simulink model "noise_suppressor"  (Simulink 7.0)
settings: Solver=FixedStepDiscrete  StartTime=0.0  StopTime=inf  RelTol=1e-3
libraries: simulink x9, dspsigops x4, dspxfrm3 x2, dspstat3 x2, dspbuff3 x1, dspwin32 x1, dspsrcs4 x1, dspsnks4 x1
settings Model: Creator=abehbood  LastModifiedBy=abehbood
settings SolverCC: PositivePriorityOrder=on
settings DataIOCC: SaveOutput=off  SaveTime=off
settings OptimizationCC: OptimizeModelRefInitCode=on
settings DebuggingCC: SaveWithParameterizedLinksMsg=none  SignalResolutionControl=TryResolveAllWithWarning  MultiTaskDSMMsg=warning  MultiTaskCondExecSysMsg=none  StrictBusMsg=None
settings HardwareCC: ProdBitPerLong=40  ProdIntDivRoundTo=Zero  ProdEndianess=LittleEndian  ProdHWDeviceType=TI C6000  TargetHWDeviceType=32-bit Generic
settings RTWCC: SystemTargetFile=ccslink_ert.tlc  GenCodeOnly=on  GenerateMakefile=off  TemplateMakefile=ccslink_ert.tmf  Description=Link for CCS (ERT) code generation for TMS320(TM) DSP platforms  ProcessScript=ccslink_ert_make_rtw_hook  IncludeERTFirstTime=on
settings CodeAppCC: IgnoreCustomStorageClasses=off
settings ERTTgtLinkCCS: TargetFcnLib=ansi_tfl_table_tmw.mat  GenFloatMathFcnCalls=ANSI_C  UtilityFuncGeneration=Auto  GenerateFullHeader=on  GenerateSampleERTMain=off  GenerateTestInterfaces=off  IsPILTarget=off  ModelReferenceCompliant=on  CompOptLevelCompliant=off  IncludeMdlTerminateFcn=on  CombineOutputUpdateFcns=on  SuppressErrorStatus=off  IncludeFileDelimiter=Auto  ERTCustomFileBanners=on  SupportAbsoluteTime=on  LogVarNameModifier=rt_  MatFileLogging=off  MultiInstanceERTCode=off  SupportNonFinite=on  SupportComplex=on  PurelyIntegerCode=off  SupportContinuousTime=off  SupportNonInlinedSFcns=off  EnableShiftOperators=on  ParenthesesLevel=Nominal  PortableWordSizes=off  ModelStepFunctionPrototypeControlCompliant=off  GenerateErtSFunction=off  GenerateASAP2=off  ExtMode=off  ExtModeTransport=0  ExtModeStaticAlloc=off  ExtModeStaticAllocSize=1000000  ExtModeTesting=off  ExtModeMexFile=ext_comm  ExtModeIntrfLevel=Level1  InlinedParameterPlacement=NonHierarchical  TargetOS=BareBoardExample  MultiInstanceErrorCode=Error  RateGroupingCode=on  RootIOFormat=Individual arguments  RTWCAPISignals=off  RTWCAPIParams=off  RTWCAPIStates=off  ERTSrcFileBannerTemplate=ert_code_template.cgt  ERTHdrFileBannerTemplate=ert_code_template.cgt  ERTDataSrcFileTemplate=ert_code_template.cgt  ERTDataHdrFileTemplate=ert_code_template.cgt  ERTCustomFileTemplate=example_file_process.tlc  ModuleNamingRule=Unspecified  SignalDisplayLevel=10  ParamTuneLevel=10  GlobalDataDefinition=Auto  DataDefinitionFile=global.c  GlobalDataReference=Auto  DataReferenceFile=global.h  GRTInterface=off  PreserveExpressionOrder=off  PreserveIfCondition=off  EnableUserReplacementTypes=off  MemSecPackage=--- None ---  MemSecDataConstants=Default  MemSecDataIO=Default  MemSecDataInternal=Default  MemSecDataParameters=Default  MemSecFuncInitTerm=Default  MemSecFuncExecute=Default  exportIDEObj=on  ideObjName=CCS_Obj  oldideObjName=CCS_Obj  ProfileGenCode=off  ProfileNumSamples=100  InlineDSPBlks=on  projectOptions=Custom  debugCompilerOptions="-g -d\"_DEBUG\""  releaseCompilerOptions=-o2  compilerOptionsStr="-o2  -q"  getCompilerOptions=off  getLinkerOptions=off  systemStackSize=8192  buildAction=Build_and_execute  overrunNotificationMethod=Print_message  overrunNotificationFcn=myfunction  oldoverrunNotificationFcn=myfunction  configurePIL=off  configPILBlockAction=Create_PIL_block_build_and_download

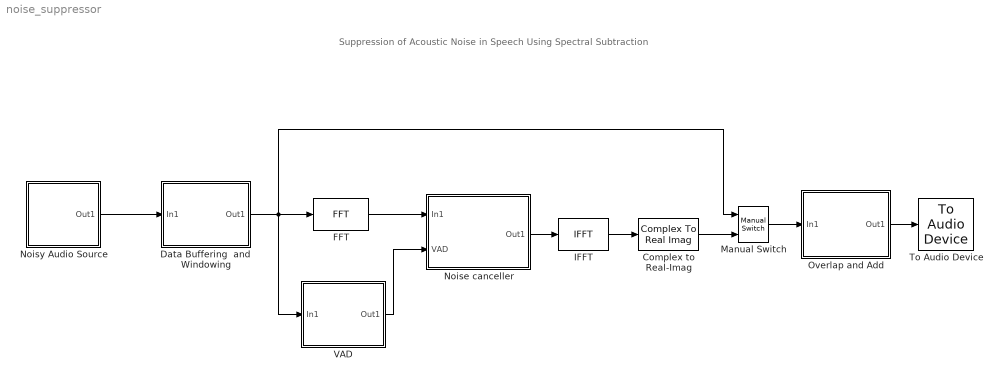
== system noise_suppressor ==
  note: Suppression of Acoustic Noise in Speech
      | Using Spectral Subtraction
  Complex to Real-Imag : ComplexToRealImag  Output=Real
  Data Buffering  and  Windowing : Subsystem
  FFT : dspxfrm3/FFT  DialogController=dspDDGCreate  DialogControllerArgs=DataTag1  CompMethod=Table lookup  TableOpt=Speed  BitRevOrder=off  InheritFFTLength=on  FFTLength=64  SkipNorm=on  roundingMode=Floor  overflowMode=off
  IFFT : dspxfrm3/IFFT  DialogController=dspDDGCreate  DialogControllerArgs=DataTag2  CompMethod=Table lookup  TableOpt=Speed  BitRevOrder=off  cs_in=off  SkipNorm=off  InheritFFTLength=on  FFTLength=64  mode=Complex  roundingMode=Floor  overflowMode=off
  Manual Switch : simulink/Signal Routing/Manual Switch  SystemSampleTime=-1  sw=0  action=0  varsize=off
  Noise canceller : Subsystem
  Noisy Audio Source : Subsystem
  Overlap and Add : Subsystem
  To Audio Device : dspsnks4/To Audio Device  DialogController=dspDDGCreate  DialogControllerArgs=DataTag6  deviceName=Default  inheritSampleRate=on  sampleRate=44100  deviceDatatype=Determine from input data type  autoBufferSize=on  bufferSize=4096  queueDuration=1.0
  VAD : Subsystem
  wires:
  Noisy Audio Source/1(Out1) -> Data Buffering  and  Windowing/1(In1)
  Overlap and Add/1(Out1) -> To Audio Device/1
  Data Buffering  and  Windowing/1(Out1) -> FFT/1, VAD/1(In1), Manual Switch/1
  FFT/1 -> Noise canceller/1(In1)
  IFFT/1 -> Complex to Real-Imag/1
  Noise canceller/1(Out1) -> IFFT/1
  VAD/1(Out1) -> Noise canceller/2(VAD)
  Manual Switch/1 -> Overlap and Add/1(In1)
  Complex to Real-Imag/1 -> Manual Switch/2

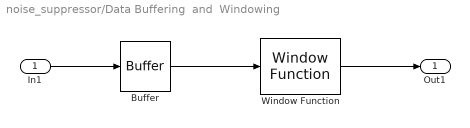
== system noise_suppressor/Data Buffering  and  Windowing ==
  In1 : Inport  OutDataType=sfix(16)  OutScaling=2^0
  Buffer : dspbuff3/Buffer  N=256  V=128  ic=0
  Window Function : dspsigops/Window Function  DialogController=dspDDGCreate  DialogControllerArgs=DataTag0  winmode=Apply window to input  wintype=Hanning  sampmode=Continuous  samptime=1  N=64  Rs=50  beta=10  winsamp=Symmetric  UserWindow=hamming  OptParams=off  UserParams={'symmetric'}  dataType=double  isSigned=on  wordLen=16  udDataType=sfix(16)  fracBitsMode=Best precision  numFracBits=15  roundingMode=Floor  overflowMode=off  numSidelobes=4  sidelobeLevel=-30
  Out1 : Outport  OutDataType=sfix(16)  OutScaling=2^0
  wires:
  Buffer/1 -> Window Function/1
  In1/1 -> Buffer/1
  Window Function/1 -> Out1/1

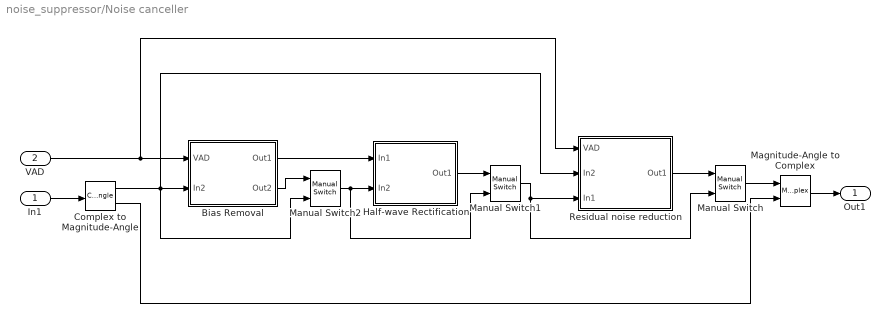
== system noise_suppressor/Noise canceller ==
  In1 : Inport  OutDataType=sfix(16)  OutScaling=2^0
  VAD : Inport  Port=2  OutDataType=sfix(16)  OutScaling=2^0
  Bias Removal : Subsystem  mask{alpha=2, beta=1.8}
  Complex to Magnitude-Angle : ComplexToMagnitudeAngle
  Half-wave Rectification : Subsystem
  Magnitude-Angle to Complex : MagnitudeAngleToComplex
  Manual Switch : simulink/Signal Routing/Manual Switch  SystemSampleTime=-1  sw=1  action=0  varsize=off
  Manual Switch1 : simulink/Signal Routing/Manual Switch  SystemSampleTime=-1  sw=1  action=0  varsize=off
  Manual Switch2 : simulink/Signal Routing/Manual Switch  SystemSampleTime=-1  sw=1  action=0  varsize=off
  Residual noise reduction : Subsystem
  Out1 : Outport  OutDataType=sfix(16)  OutScaling=2^0
  wires:
  In1/1 -> Complex to Magnitude-Angle/1
  Magnitude-Angle to Complex/1 -> Out1/1
  Complex to Magnitude-Angle/2 -> Magnitude-Angle to Complex/2
  VAD/1 -> Bias Removal/1(VAD), Residual noise reduction/1(VAD)
  Residual noise reduction/1(Out1) -> Manual Switch/1
  Half-wave Rectification/1(Out1) -> Manual Switch1/1
  Manual Switch2/1 -> Manual Switch1/2, Half-wave Rectification/2(In2)
  Complex to Magnitude-Angle/1 -> Bias Removal/2(In2), Manual Switch2/2, Residual noise reduction/2(In2)
  Bias Removal/1(Out1) -> Half-wave Rectification/1(In1)
  Bias Removal/2(Out2) -> Manual Switch2/1
  Manual Switch/1 -> Magnitude-Angle to Complex/1
  Manual Switch1/1 -> Residual noise reduction/3(In1), Manual Switch/2

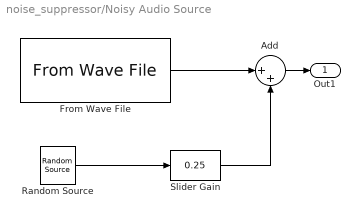
== system noise_suppressor/Noisy Audio Source ==
  Add : Sum  Inputs=|++  OutDataType=sfix(16)  OutScaling=2^-10
  From Wave File : dspwin32/From Wave File  FileName=speech_dft_8k_2.wav  SamplesPerFrame=256  MinBufSize=1  dType=single  bLoop=on  timesToPlay=10  restartMode=immediately after last sample  firstSampleOutput=off  lastSampleOutput=off
  Random Source : dspsrcs4/Random Source  SrcType=Uniform  NormMethod=Ziggurat  CltLength=12  MinVal=-.05  MaxVal=.05  MeanVal=0  VarVal=1  RepMode=Not repeatable  rawSeed=1  IsInherit=off  SampMode=Discrete  SampTime=-1  SampFrame=256  DataType=Single  OutComplex=Real
  Slider Gain : simulink/Math Operations/Slider Gain  SystemSampleTime=-1  low=0  gain=0.25  high=1
  Out1 : Outport  OutDataType=sfix(16)  OutScaling=2^0
  wires:
  Add/1 -> Out1/1
  Slider Gain/1 -> Add/2
  Random Source/1 -> Slider Gain/1
  From Wave File/1 -> Add/1

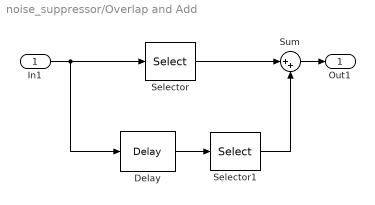
== system noise_suppressor/Overlap and Add ==
  In1 : Inport  OutDataType=sfix(16)  OutScaling=2^0
  Delay : dspsigops/Delay  dly_unit=Frames  delay=1  ic_detail=off  dif_ic_for_ch=off  dif_ic_for_dly=off  ic=0  reset_popup=None
  Selector : Selector  InputPortWidth=256  IndexOptions=Index vector (dialog)  Indices=1:128  OutputSizes=1
  Selector1 : Selector  InputPortWidth=256  IndexOptions=Index vector (dialog)  Indices=129:256  OutputSizes=1
  Sum : Sum  Inputs=|++  OutDataType=sfix(16)  OutScaling=2^0
  Out1 : Outport  OutDataType=sfix(16)  OutScaling=2^0
  wires:
  Selector/1 -> Sum/1
  Delay/1 -> Selector1/1
  Selector1/1 -> Sum/2
  In1/1 -> Delay/1, Selector/1
  Sum/1 -> Out1/1

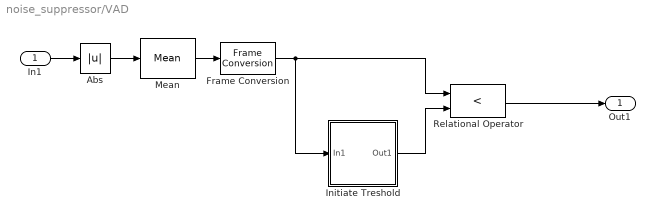
== system noise_suppressor/VAD ==
  In1 : Inport  OutDataType=sfix(16)  OutScaling=2^0
  Abs : Abs
  Frame Conversion : FrameConversion  OutFrame=Sample based
  Initiate Treshold : Subsystem
  Mean : dspstat3/Mean  DialogController=dspDDGCreate  DialogControllerArgs=DataTag7  run=off  reset_popup=None  roundingMode=Floor  overflowMode=off
  Relational Operator : RelationalOperator  Operator=<  LogicOutDataTypeMode=boolean
  Out1 : Outport  OutDataType=sfix(16)  OutScaling=2^0
  wires:
  Abs/1 -> Mean/1
  Mean/1 -> Frame Conversion/1
  Initiate Treshold/1(Out1) -> Relational Operator/2
  Relational Operator/1 -> Out1/1
  In1/1 -> Abs/1
  Frame Conversion/1 -> Initiate Treshold/1(In1), Relational Operator/1

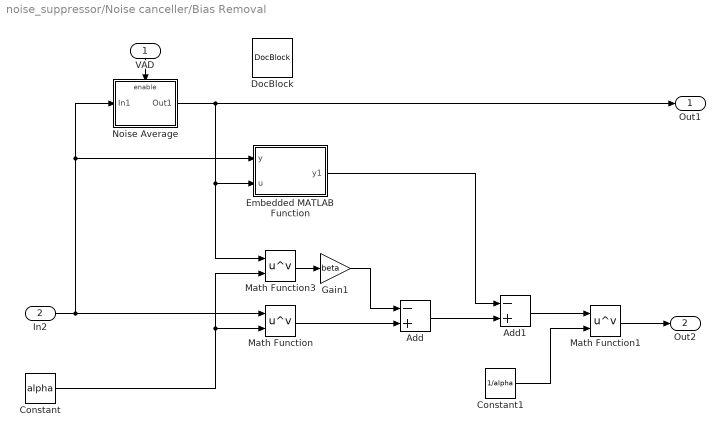
== system noise_suppressor/Noise canceller/Bias Removal ==
  VAD : Inport  Orientation=down  OutDataType=sfix(16)  OutScaling=2^0
  In2 : Inport  Port=2  OutDataType=sfix(16)  OutScaling=2^0
  Add : Sum  Inputs=-+  OutDataType=sfix(16)  OutScaling=2^-10
  Add1 : Sum  Inputs=-+  OutDataType=sfix(16)  OutScaling=2^-10
  Constant : Constant  Value=alpha  OutDataType=sfix(16)  OutScaling=2^0
  Constant1 : Constant  Value=1/alpha  OutDataType=sfix(16)  OutScaling=2^0
  DocBlock : simulink/Model-Wide Utilities/DocBlock  SystemSampleTime=-1  DocumentType=Text
  Embedded MATLAB Function : Stateflow chart
  Gain1 : Gain  Gain=beta  ParameterDataType=sfix(16)  ParameterScaling=2^0  OutDataType=sfix(16)  OutScaling=2^0
  Math Function : Math  Operator=pow  OutDataType=sfix(16)  OutScaling=2^0  SaturateOnIntegerOverflow=on
  Math Function1 : Math  Operator=pow  OutDataType=sfix(16)  OutScaling=2^0  SaturateOnIntegerOverflow=on
  Math Function3 : Math  Operator=pow  OutDataType=sfix(16)  OutScaling=2^0  SaturateOnIntegerOverflow=on
  Noise Average : Subsystem  TreatAsAtomicUnit=on
  Out1 : Outport  OutDataType=sfix(16)  OutScaling=2^0
  Out2 : Outport  Port=2  OutDataType=sfix(16)  OutScaling=2^0
  wires:
  In2/1 -> Math Function/1, Noise Average/1(In1), Embedded MATLAB Function/1(y)
  VAD/1 -> Noise Average/Enable
  Math Function1/1 -> Out2/1
  Constant/1 -> Math Function/2, Math Function3/2
  Constant1/1 -> Math Function1/2
  Math Function/1 -> Add/2
  Gain1/1 -> Add/1
  Noise Average/1(Out1) -> Math Function3/1, Embedded MATLAB Function/2(u), Out1/1
  Add1/1 -> Math Function1/1
  Math Function3/1 -> Gain1/1
  Add/1 -> Add1/2
  Embedded MATLAB Function/1(y1) -> Add1/1

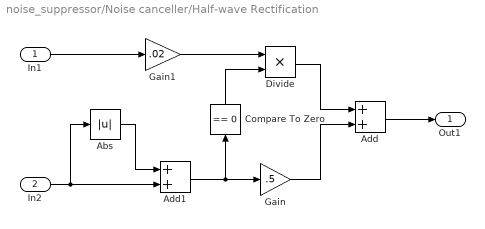
== system noise_suppressor/Noise canceller/Half-wave Rectification ==
  In1 : Inport  OutDataType=sfix(16)  OutScaling=2^0
  In2 : Inport  Port=2  OutDataType=sfix(16)  OutScaling=2^0
  Abs : Abs
  Add : Sum  OutDataType=sfix(16)  OutScaling=2^-10
  Add1 : Sum  OutDataType=sfix(16)  OutScaling=2^-10
  Compare To Zero : simulink/Logic and Bit Operations/Compare To Zero  Orientation=up  SystemSampleTime=-1  relop===  LogicOutDataTypeMode=uint8  ZeroCross=off
  Divide : Product  Inputs=**  OutDataType=sfix(16)  OutScaling=2^-10
  Gain : Gain  Gain=.5  ParameterDataType=sfix(16)  ParameterScaling=2^0  OutDataType=sfix(16)  OutScaling=2^0
  Gain1 : Gain  Gain=.02  ParameterDataType=sfix(16)  ParameterScaling=2^0  OutDataType=sfix(16)  OutScaling=2^0
  Out1 : Outport  OutDataType=sfix(16)  OutScaling=2^0
  wires:
  In2/1 -> Add1/2, Abs/1
  Add1/1 -> Gain/1, Compare To Zero/1
  Abs/1 -> Add1/1
  Gain/1 -> Add/2
  Add/1 -> Out1/1
  In1/1 -> Gain1/1
  Compare To Zero/1 -> Divide/2
  Divide/1 -> Add/1
  Gain1/1 -> Divide/1

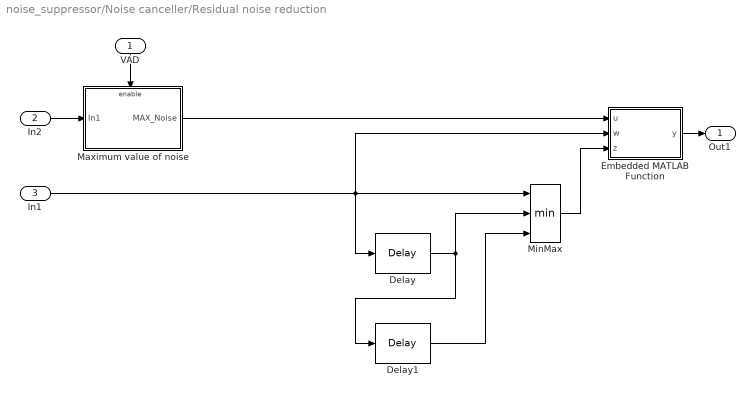
== system noise_suppressor/Noise canceller/Residual noise reduction ==
  VAD : Inport  Orientation=down  OutDataType=sfix(16)  OutScaling=2^0
  In2 : Inport  Port=2  OutDataType=sfix(16)  OutScaling=2^0
  In1 : Inport  Port=3  OutDataType=sfix(16)  OutScaling=2^0
  Delay : dspsigops/Delay  dly_unit=Samples  delay=1  ic_detail=off  dif_ic_for_ch=off  dif_ic_for_dly=off  ic=0  reset_popup=None
  Delay1 : dspsigops/Delay  dly_unit=Samples  delay=1  ic_detail=off  dif_ic_for_ch=off  dif_ic_for_dly=off  ic=0  reset_popup=None
  Embedded MATLAB Function : Stateflow chart
  Maximum value of noise : Subsystem  TreatAsAtomicUnit=on
  MinMax : MinMax  Inputs=3  OutDataType=sfix(16)  OutScaling=2^0
  Out1 : Outport  OutDataType=sfix(16)  OutScaling=2^0
  wires:
  Delay/1 -> Delay1/1, MinMax/2
  Delay1/1 -> MinMax/3
  Maximum value of noise/1(MAX_Noise) -> Embedded MATLAB Function/1(u)
  MinMax/1 -> Embedded MATLAB Function/3(z)
  VAD/1 -> Maximum value of noise/Enable
  In2/1 -> Maximum value of noise/1(In1)
  Embedded MATLAB Function/1(y) -> Out1/1
  In1/1 -> MinMax/1, Delay/1, Embedded MATLAB Function/2(w)

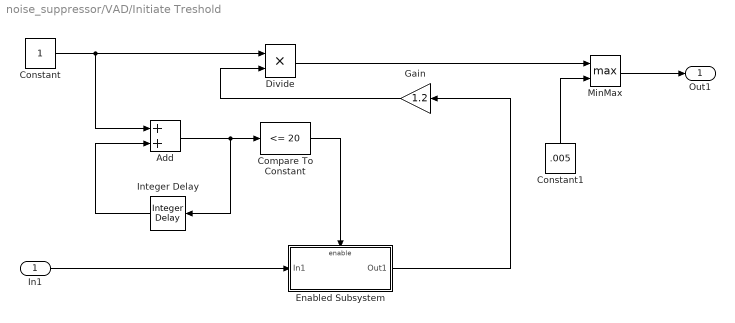
== system noise_suppressor/VAD/Initiate Treshold ==
  In1 : Inport  OutDataType=sfix(16)  OutScaling=2^0
  Add : Sum  OutDataType=sfix(16)  OutScaling=2^-10
  Compare To Constant : simulink/Logic and Bit Operations/Compare To Constant  SystemSampleTime=-1  relop=<=  const=20  LogicOutDataTypeMode=boolean  ZeroCross=off
  Constant : Constant  OutDataType=sfix(16)  OutScaling=2^0  SampleTime=-1
  Constant1 : Constant  Orientation=up  Value=.005  OutDataType=sfix(16)  OutScaling=2^0  SampleTime=-1
  Divide : Product  Inputs=**  OutDataType=sfix(16)  OutScaling=2^-10
  Enabled Subsystem : Subsystem  TreatAsAtomicUnit=on
  Gain : Gain  Orientation=left  Gain=1.2  ParameterDataType=sfix(16)  ParameterScalingMode=Use specified scaling  ParameterScaling=2^-14  OutDataType=sfix(16)  OutScaling=2^0
  Integer Delay : simulink/Discrete/Integer Delay  Orientation=left  vinit=0.0  samptime=-1  NumDelays=1
  MinMax : MinMax  Function=max  Inputs=2  OutDataType=sfix(16)  OutScaling=2^0
  Out1 : Outport  OutDataType=sfix(16)  OutScaling=2^0
  wires:
  Constant/1 -> Add/1, Divide/1
  Integer Delay/1 -> Add/2
  Add/1 -> Integer Delay/1, Compare To Constant/1
  Compare To Constant/1 -> Enabled Subsystem/Enable
  Enabled Subsystem/1(Out1) -> Gain/1
  Gain/1 -> Divide/2
  In1/1 -> Enabled Subsystem/1(In1)
  Divide/1 -> MinMax/1
  MinMax/1 -> Out1/1
  Constant1/1 -> MinMax/2

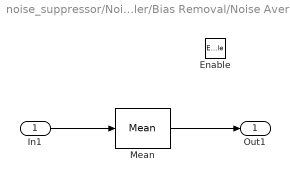
== system noise_suppressor/Noise canceller/Bias Removal/Noise Average ==
  In1 : Inport  OutDataType=sfix(16)  OutScaling=2^0
  Enable : EnablePort
  Mean : dspstat3/Mean  DialogController=dspDDGCreate  DialogControllerArgs=DataTag4  run=on  reset_popup=None  roundingMode=Floor  overflowMode=off
  Out1 : Outport  OutDataType=sfix(16)  OutScaling=2^0
  wires:
  In1/1 -> Mean/1
  Mean/1 -> Out1/1

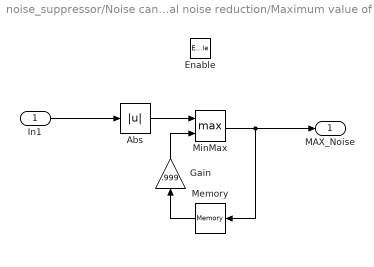
== system noise_suppressor/Noise canceller/Residual noise reduction/Maximum value of noise ==
  In1 : Inport  OutDataType=sfix(16)  OutScaling=2^0
  Enable : EnablePort
  Abs : Abs
  Gain : Gain  Orientation=up  Gain=.999  ParameterDataType=sfix(16)  ParameterScaling=2^0  OutDataType=sfix(16)  OutScaling=2^0
  Memory : Memory  Orientation=left  InheritSampleTime=on
  MinMax : MinMax  Function=max  Inputs=2  OutDataType=sfix(16)  OutScaling=2^0
  MAX_Noise : Outport  OutDataType=sfix(16)  OutScaling=2^0
  wires:
  MinMax/1 -> MAX_Noise/1, Memory/1
  Memory/1 -> Gain/1
  Gain/1 -> MinMax/2
  Abs/1 -> MinMax/1
  In1/1 -> Abs/1

== system noise_suppressor/VAD/Initiate Treshold/Enabled Subsystem ==
  In1 : Inport  OutDataType=sfix(16)  OutScaling=2^0
  Enable : EnablePort
  Out1 : Outport  OutDataType=sfix(16)  OutScaling=2^0
  wires:
  In1/1 -> Out1/1

== matlab function Noise canceller/Bias Removal/Embedded MATLAB Function ==
  data: y input inherited; u input inherited; y1 output inherited
function y1  = fcn(y,u)
% This block supports an embeddable subset of the MATLAB language.
% See the help menu for details. 

my = mean(y);
mu = mean(u);

vary=mean((y-my).^2);
varu=mean((u-mu).^2);

covyv=mean(abs((y-my).*(u-mu)));

g=covyv/sqrt(vary*varu);

y1=y.*u*g;

== matlab function Noise canceller/Residual noise reduction/Embedded MATLAB Function ==
  data: u input inherited; y output inherited; w input inherited; z input inherited
function y = fcn(u,w,z)
% This block supports an embeddable subset of the MATLAB language.
% See the help menu for details. 


y = w;

for i=1:256;
    if (w(i)<u(i))
        y(i)=z(i);
    end
end
